simulink model "cosimulink"  (Simulink 9.1)
settings: Solver=VariableStepAuto  StartTime=0.0  StopTime=60  RelTol=1e-3
libraries: Solver_SF x1
settings Model: Creator=Administrator  LastModifiedBy=Administrator
settings DataIOCC: SaveFormat=Dataset
settings OptimizationCC: LifeSpan=auto
settings DebuggingCC: UnderspecifiedInitializationDetection=Simplified  MergeDetectMultiDrivingBlocksExec=error  SFUnexpectedBacktrackingDiag=error  SFNoUnconditionalDefaultTransitionDiag=error  SFExecutionAtInitializationDiag=warning
settings HardwareCC: ProdBitPerPointer=64  ProdBitPerSizeT=64  ProdBitPerPtrDiffT=64  ProdLargestAtomicFloat=Float  ProdIntDivRoundTo=Zero  ProdEndianess=LittleEndian  ProdWordSize=64  ProdHWDeviceType=Intel->x86-64 (Windows64)
settings ModelReferenceCC: PropagateSignalLabelsOutOfModel=on
settings CodeAppCC: StateflowObjectComments=off
settings GRTTargetCC: TargetLangStandard=C99 (ISO)  CombineOutputUpdateFcns=on  GRTInterface=off
settings ConfigComp: CovMetricSettings=dwe  CovHtmlReporting=off  CovSaveCumulativeToWorkspaceVar=off  CovSaveSingleToWorkspaceVar=off  CovExternalEMLEnable=on

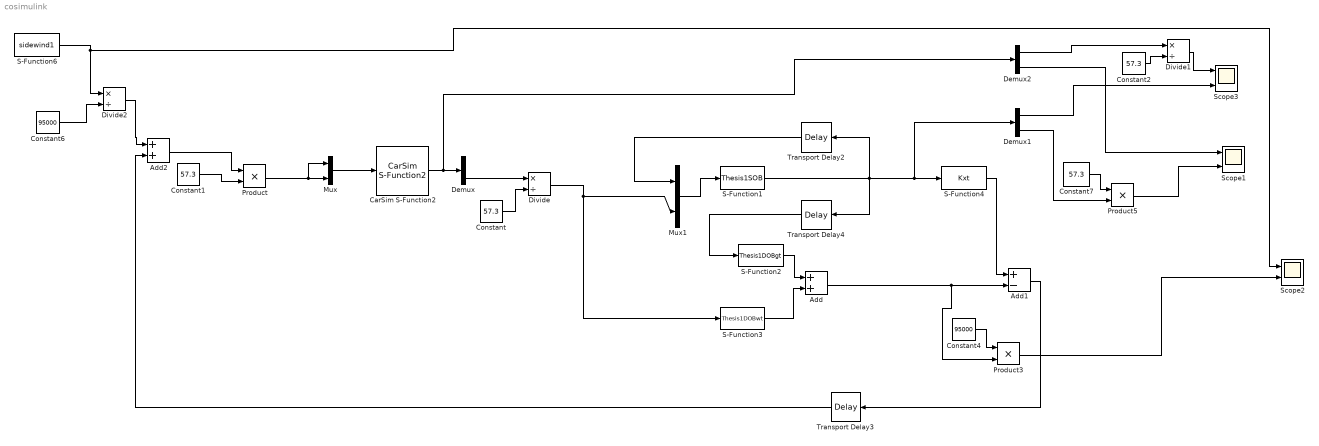
== system cosimulink ==
  Add : Sum
  Add1 : Sum  Inputs=+-
  Add2 : Sum
  CarSim S-Function2 : Solver_SF/CarSim S-Function2  Priority=1  VehicleCode=i_i  SIMFILE=simfile.sim
      settings: AttributesFormatString=Vehicle Code: %<VehicleCode>
  Constant{,1..2,7} (4 alike) : Constant  Value=57.3
  Constant4 : Constant  Value=95000
  Constant6 : Constant  Value=95000
  Demux : Demux  Outputs=2
  Demux1 : Demux  Outputs=2
  Demux2 : Demux  Outputs=2
  Divide : Product  Inputs=*/
  Divide1 : Product  Inputs=*/
  Divide2 : Product  Inputs=*/
  Mux : Mux  Inputs=2
  Mux1 : Mux  Inputs=2
  Product : Product
  Product3 : Product
  Product5 : Product
  S-Function1 : S-Function  FunctionName=Thesis1SOB  SFunctionDeploymentMode=off  EnableBusSupport=off
  S-Function2 : S-Function  FunctionName=Thesis1DOBgt  SFunctionDeploymentMode=off  EnableBusSupport=off
  S-Function3 : S-Function  FunctionName=Thesis1DOBwt  SFunctionDeploymentMode=off  EnableBusSupport=off
  S-Function4 : S-Function  FunctionName=Kxt  SFunctionDeploymentMode=off  EnableBusSupport=off
  S-Function6 : S-Function  FunctionName=sidewind1  SFunctionDeploymentMode=off  EnableBusSupport=off
  Scope1 : Scope  NumInputPorts=2
  Scope2 : Scope  NumInputPorts=2
  Scope3 : Scope  NumInputPorts=2
  Transport Delay2 : TransportDelay  DelayTime=0.019
  Transport Delay3 : TransportDelay  DelayTime=0.019
  Transport Delay4 : TransportDelay  DelayTime=0.019
  wires:
  Constant/1 -> Divide/2
  Demux/2 -> Divide/1
  Divide/1 -> S-Function3/1, Mux1/2
  Mux1/1 -> S-Function1/1
  S-Function2/1 -> Add/1
  S-Function3/1 -> Add/2
  S-Function4/1 -> Add1/1
  Add/1 -> Product3/2, Add1/2
  Divide2/1 -> Add2/1
  S-Function1/1 -> Demux1/1, S-Function4/1, Transport Delay2/1, Transport Delay4/1
  Constant4/1 -> Product3/1
  Product3/1 -> Scope2/2
  Constant1/1 -> Product/2
  Mux/1 -> CarSim S-Function2/1
  Constant6/1 -> Divide2/2
  S-Function6/1 -> Scope2/1, Divide2/1
  Add2/1 -> Product/1
  Constant7/1 -> Product5/1
  Demux1/2 -> Product5/2
  Add1/1 -> Transport Delay3/1
  Product/1 -> Mux/2, Mux/1
  Transport Delay2/1 -> Mux1/1
  Constant2/1 -> Divide1/2
  CarSim S-Function2/1 -> Demux2/1, Demux/1
  Demux2/1 -> Divide1/1
  Divide1/1 -> Scope3/1
  Demux1/1 -> Scope3/2
  Product5/1 -> Scope1/2
  Demux2/2 -> Scope1/1
  Transport Delay4/1 -> S-Function2/1
  Transport Delay3/1 -> Add2/2
